simulink model "PV_module"  (Simulink 8.4)
settings: Solver=FixedStepDiscrete  StartTime=0.0  StopTime=1  FixedStep=1e-4  RelTol=1e-3
libraries: simulink x1
settings Model: Creator=amaki  LastModifiedBy=lappalak
settings DebuggingCC: AlgebraicLoopMsg=none
settings ConfigurationSet: Description=SimMechanics 2G

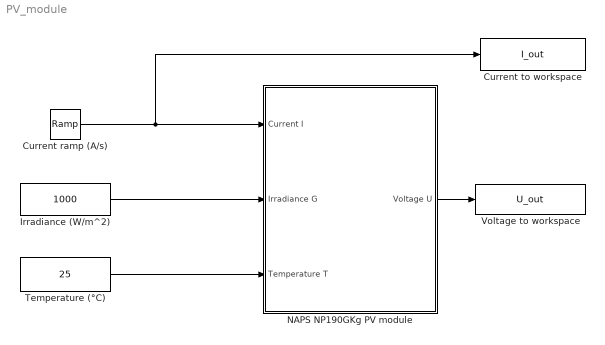
== system PV_module ==
  Current ramp (A/s) : simulink/Sources/Ramp  slope=10  start=0  X0=0
  Current to workspace : ToWorkspace  VariableName=I_out  SampleTime=-1
  Irradiance (W/m^2) : Constant  Value=1000
  NAPS NP190GKg PV module : Subsystem  mask{Isc_stc=8.02, Uoc_stc=33.1, G_stc=1000, T_stc=273.15+25, Ns=54, Rs=0.33, Rsh=188, A=1.3, Ku=-0.1242, Ki=0.0047, k=1.3806503e-23, q=1.60217646e-19}
      mask prompts: Isc_stc "STC short-circuit current"; Uoc_stc "STC open-circuit voltage"; G_stc "STC irradiance"; T_stc "STC temperature"; Ns "Number of cells"; Rs "Series resistance Rs"; Rsh "Shunt resistance Rsh"; A "Ideality factor A"; Ku "Temp. coeff. of OC Ku"; Ki "Temp. coeff. of SC Ki"; k "Boltzmann constant"; q "Elementary charge"
  Temperature (°C) : Constant  Value=25
  Voltage to workspace : ToWorkspace  VariableName=U_out  SampleTime=-1
  wires:
  Current ramp (A/s)/1 -> Current to workspace/1, NAPS NP190GKg PV module/1(Current I)
  Irradiance (W/m^2)/1 -> NAPS NP190GKg PV module/2(Irradiance G)
  Temperature (°C)/1 -> NAPS NP190GKg PV module/3(Temperature T)
  NAPS NP190GKg PV module/1(Voltage U) -> Voltage to workspace/1

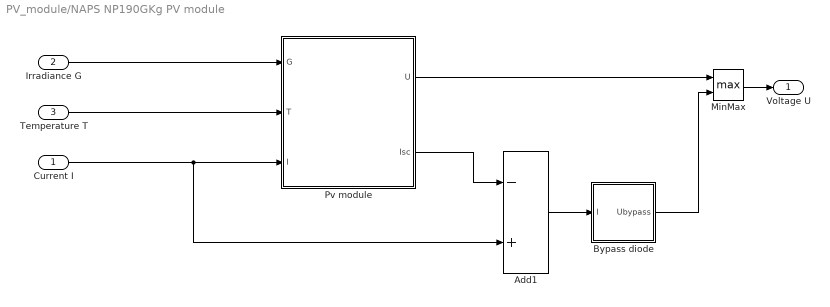
== system PV_module/NAPS NP190GKg PV module ==
  Current I : Inport
  Irradiance G : Inport  Port=2
  Temperature T : Inport  Port=3
  Add1 : Sum  Inputs=-+
  Bypass diode : Subsystem  mask{k=1.3806503e-23, q=1.60217646e-19, Rs_bypass=0.02}
      mask prompts: k "Boltzmann constant"; q "Elementary charge"; Rs_bypass "Series resistance"
  MinMax : MinMax  Function=max  Inputs=2
  Pv module : Subsystem
  Voltage U : Outport
  wires:
  MinMax/1 -> Voltage U/1
  Add1/1 -> Bypass diode/1(I)
  Bypass diode/1(Ubypass) -> MinMax/2
  Pv module/2(Isc) -> Add1/1
  Pv module/1(U) -> MinMax/1
  Irradiance G/1 -> Pv module/1(G)
  Temperature T/1 -> Pv module/2(T)
  Current I/1 -> Pv module/3(I), Add1/2

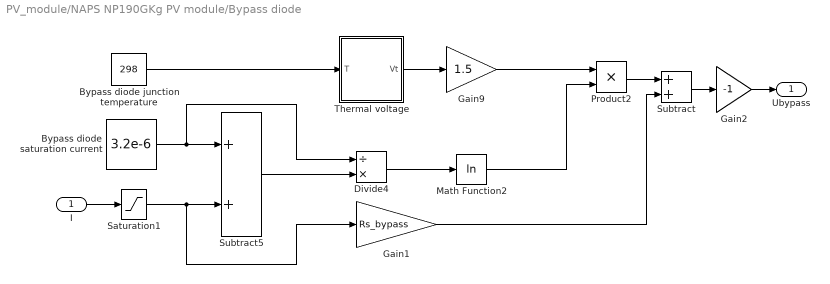
== system PV_module/NAPS NP190GKg PV module/Bypass diode ==
  I : Inport
  Bypass diode junction temperature : Constant  Value=298
  Bypass diode saturation current : Constant  Value=3.2e-6
  Divide4 : Product  Inputs=/*
  Gain1 : Gain  Gain=Rs_bypass
  Gain2 : Gain  Gain=-1
  Gain9 : Gain  Gain=1.5
  Math Function2 : Math  Operator=log  SaturateOnIntegerOverflow=on
  Product2 : Product  RndMeth=Zero
  Saturation1 : Saturate  UpperLimit=1e24  LowerLimit=0
  Subtract : Sum
  Subtract5 : Sum
  Thermal voltage : Subsystem
  Ubypass : Outport
  wires:
  Gain2/1 -> Ubypass/1
  Subtract/1 -> Gain2/1
  Saturation1/1 -> Gain1/1, Subtract5/2
  Subtract5/1 -> Divide4/2
  Divide4/1 -> Math Function2/1
  Bypass diode junction temperature/1 -> Thermal voltage/1(T)
  Gain1/1 -> Subtract/2
  Product2/1 -> Subtract/1
  I/1 -> Saturation1/1
  Bypass diode saturation current/1 -> Divide4/1, Subtract5/1
  Thermal voltage/1(Vt) -> Gain9/1
  Gain9/1 -> Product2/1
  Math Function2/1 -> Product2/2

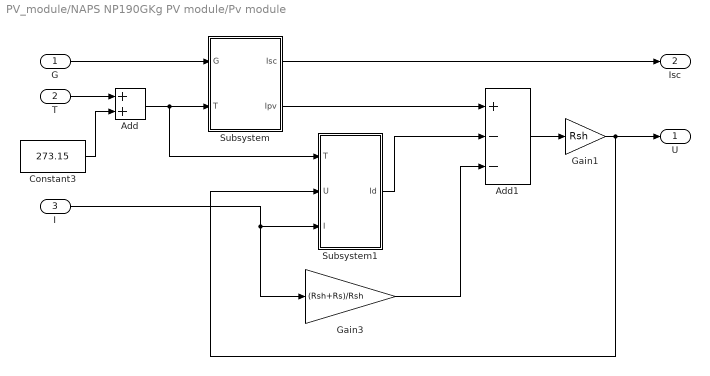
== system PV_module/NAPS NP190GKg PV module/Pv module ==
  G : Inport
  T : Inport  Port=2
  I : Inport  Port=3
  Add : Sum
  Add1 : Sum  Inputs=+--
  Constant3 : Constant  Value=273.15
  Gain1 : Gain  Gain=Rsh
  Gain3 : Gain  Gain=(Rsh+Rs)/Rsh
  Subsystem : Subsystem
  Subsystem1 : Subsystem
  U : Outport
  Isc : Outport  Port=2
  wires:
  Subsystem/1(Isc) -> Isc/1
  Gain1/1 -> Subsystem1/2(U), U/1
  Add1/1 -> Gain1/1
  Gain3/1 -> Add1/3
  I/1 -> Gain3/1, Subsystem1/3(I)
  Subsystem1/1(Id) -> Add1/2
  G/1 -> Subsystem/1(G)
  Subsystem/2(Ipv) -> Add1/1
  Constant3/1 -> Add/2
  Add/1 -> Subsystem1/1(T), Subsystem/2(T)
  T/1 -> Add/1

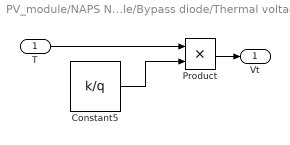
== system PV_module/NAPS NP190GKg PV module/Bypass diode/Thermal voltage ==
  T : Inport
  Constant5 : Constant  Value=k/q
  Product : Product  RndMeth=Zero
  Vt : Outport
  wires:
  Product/1 -> Vt/1
  T/1 -> Product/1
  Constant5/1 -> Product/2

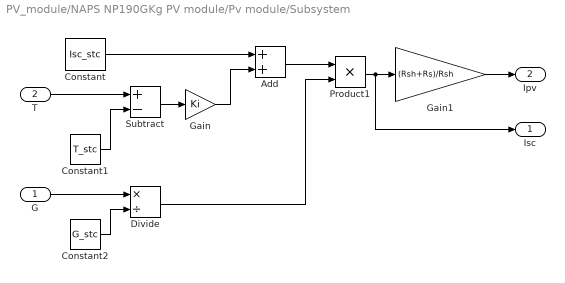
== system PV_module/NAPS NP190GKg PV module/Pv module/Subsystem ==
  G : Inport
  T : Inport  Port=2
  Add : Sum
  Constant : Constant  Value=Isc_stc
  Constant1 : Constant  Value=T_stc
  Constant2 : Constant  Value=G_stc
  Divide : Product  Inputs=*/
  Gain : Gain  Gain=Ki
  Gain1 : Gain  Gain=(Rsh+Rs)/Rsh
  Product1 : Product  RndMeth=Zero
  Subtract : Sum  Inputs=+-
  Isc : Outport
  Ipv : Outport  Port=2
  wires:
  Gain1/1 -> Ipv/1
  Product1/1 -> Isc/1, Gain1/1
  Divide/1 -> Product1/2
  Add/1 -> Product1/1
  G/1 -> Divide/1
  T/1 -> Subtract/1
  Constant2/1 -> Divide/2
  Subtract/1 -> Gain/1
  Constant1/1 -> Subtract/2
  Gain/1 -> Add/2
  Constant/1 -> Add/1

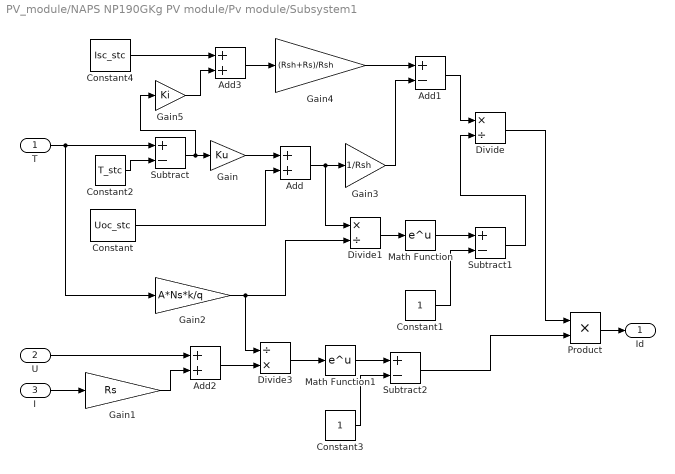
== system PV_module/NAPS NP190GKg PV module/Pv module/Subsystem1 ==
  T : Inport
  U : Inport  Port=2
  I : Inport  Port=3
  Add : Sum
  Add1 : Sum  Inputs=+-
  Add2 : Sum
  Add3 : Sum
  Constant : Constant  Value=Uoc_stc
  Constant1 : Constant
  Constant2 : Constant  Value=T_stc
  Constant3 : Constant
  Constant4 : Constant  Value=Isc_stc
  Divide : Product  Inputs=*/
  Divide1 : Product  Inputs=*/
  Divide3 : Product  Inputs=/*
  Gain : Gain  Gain=Ku
  Gain1 : Gain  Gain=Rs
  Gain2 : Gain  Gain=A*Ns*k/q
  Gain3 : Gain  Gain=1/Rsh
  Gain4 : Gain  Gain=(Rsh+Rs)/Rsh
  Gain5 : Gain  Gain=Ki
  Math Function : Math  SaturateOnIntegerOverflow=on
  Math Function1 : Math  SaturateOnIntegerOverflow=on
  Product : Product  RndMeth=Zero
  Subtract : Sum  Inputs=+-
  Subtract1 : Sum  Inputs=+-
  Subtract2 : Sum  Inputs=+-
  Id : Outport
  wires:
  Gain4/1 -> Add1/1
  Subtract/1 -> Gain5/1, Gain/1
  Constant/1 -> Add/2
  Gain/1 -> Add/1
  Add3/1 -> Gain4/1
  Gain5/1 -> Add3/2
  Gain3/1 -> Add1/2
  Gain1/1 -> Add2/2
  I/1 -> Gain1/1
  Add/1 -> Gain3/1, Divide1/1
  Product/1 -> Id/1
  Subtract2/1 -> Product/2
  Constant3/1 -> Subtract2/2
  Math Function1/1 -> Subtract2/1
  Divide3/1 -> Math Function1/1
  Add2/1 -> Divide3/2
  U/1 -> Add2/1
  Divide/1 -> Product/1
  Subtract1/1 -> Divide/2
  Math Function/1 -> Subtract1/1
  Divide1/1 -> Math Function/1
  Gain2/1 -> Divide3/1, Divide1/2
  Constant1/1 -> Subtract1/2
  Add1/1 -> Divide/1
  T/1 -> Gain2/1, Subtract/1
  Constant2/1 -> Subtract/2
  Constant4/1 -> Add3/1
